simulink model "diagramaBloques"  (R2024b)
settings: Solver=VariableStepAuto  StartTime=0.0  StopTime=10.0  RelTol=1e-3
settings Model: Creator=estel  LastModifiedBy=estel

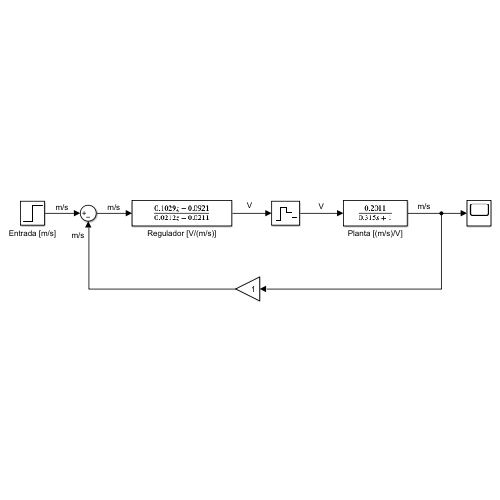
[thumbnail: Simulink's stored preview of the top-level diagram]
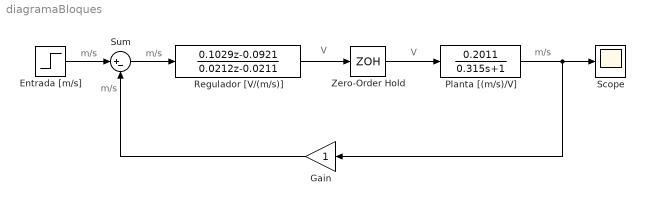
== system diagramaBloques ==
  note: m/s
  note: m/s
  note: m/s
  note: m/s
  note: V
  note: V
  Entrada [m/s] : Step  SampleTime=0
  Gain : Gain
  Planta [(m/s)/V] : TransferFcn  Numerator=[0.2011]  Denominator=[0.315 1]
  Regulador [V/(m/s)] : DiscreteTransferFcn  Numerator=[0.1029 -0.0921]  Denominator=[0.0212 -0.0211]
  Scope : Scope
  Sum : Sum  Inputs=|+-
  Zero-Order Hold : ZeroOrderHold  SampleTime=-1
  wires:
  Entrada [m/s]/1 -> Sum/1
  Sum/1 -> Regulador [V/(m/s)]/1
  Regulador [V/(m/s)]/1 -> Zero-Order Hold/1
  Zero-Order Hold/1 -> Planta [(m/s)/V]/1
  Planta [(m/s)/V]/1 -> Gain/1, Scope/1
  Gain/1 -> Sum/2
